simulink model "model"  (R2023b)
settings: Solver=VariableStepAuto  StartTime=0.0  StopTime=100.0  RelTol=1e-3
values from neighbouring files (symbols this model uses):
  a = 0.01    [parametry.m]
  k = 0.5    [parametry.m]
  m = 1    [parametry.m]
  x_0 = 0.5    [parametry.m]
  x_prim_0 = 0    [parametry.m]
settings Model: Creator=student  LastModifiedBy=Jakub

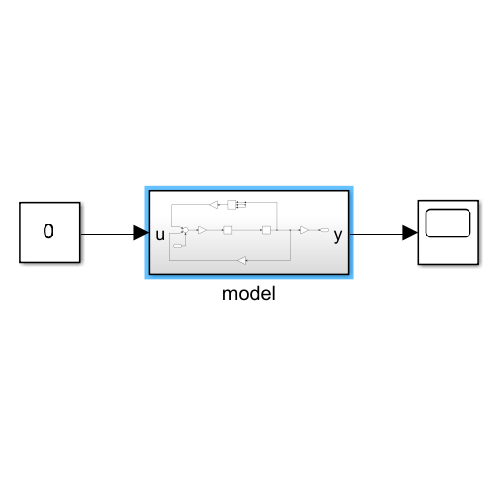
[thumbnail: Simulink's stored preview of the top-level diagram]
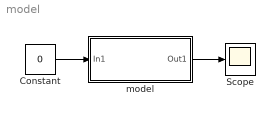
== system model ==
  Constant : Constant  Value=0
  Scope : Scope
  model : Subsystem
  wires:
  model/1(Out1) -> Scope/1
  Constant/1 -> model/1(In1)

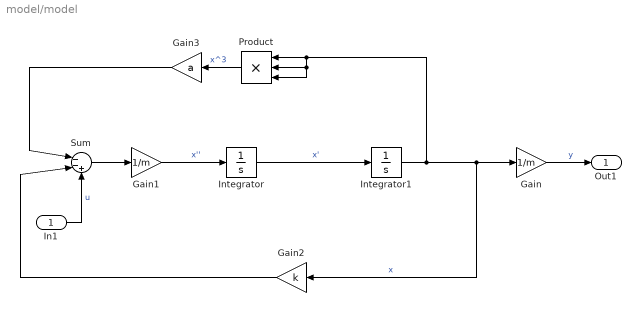
== system model/model ==
  In1 : Inport
  Gain : Gain  Gain=1/m
  Gain1 : Gain  Gain=1/m
  Gain2 : Gain  Gain=k
  Gain3 : Gain  Gain=a
  Integrator : Integrator  InitialCondition=x_prim_0
  Integrator1 : Integrator  InitialCondition=x_0
  Product : Product  Inputs=3
  Sum : Sum  Inputs=|--+
  Out1 : Outport
  wires:
  Gain1/1 -> Integrator/1  "x''"
  Integrator/1 -> Integrator1/1  "x'"
  Integrator1/1 -> Product/3, Product/2, Product/1, Gain2/1, Gain/1  "x"
  Gain/1 -> Out1/1  "y"
  Sum/1 -> Gain1/1
  Gain2/1 -> Sum/2
  Product/1 -> Gain3/1  "x^3"
  Gain3/1 -> Sum/1
  In1/1 -> Sum/3  "u"
